simulink model "StateMachine2018b"  (R2018b)
settings: Solver=VariableStepAuto  StartTime=0.0  StopTime=10.0  RelTol=1e-3
settings Model: Creator=lenovo  LastModifiedBy=lenovo
settings DataIOCC: ReturnWorkspaceOutputs=on

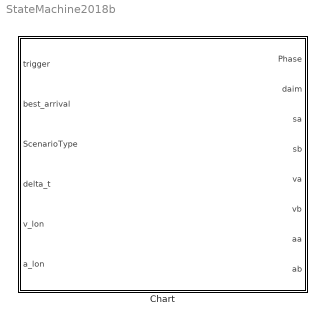
== system StateMachine2018b ==
  Chart : Stateflow chart  TreatAsAtomicUnit=on

== stateflow chart StateMachine2018b/Chart ==
  state initial
    en:
    sa = 0;
    sb = 40;
    va = 40/3.6;
    vb = 40/3.6;
    aa = 0;
    ab = 0;
    daim = 0;
    Phase = 0;
    du:
    Phase = 0;
    daim = 0;
    if (ScenarioType == 1)
    sa = 0;
    sb = 40;
    va = 40/3.6;
    vb = 40/3.6;
    aa = 0;
    ab = 0;
    else
    sa = -40;
    sb = 0;
    va = 40/3.6;
    vb = 40/3.6;
    aa = 0;
    ab = 0;
    end
  state phase1
    du:
    Phase = 1;
    sa = sa + delta_t * (va - v_lon) + 1/2 * (aa-a_lon) * delta_t^2;
    va = va + delta_t * aa;
    aa = 0;
    sb = sb + delta_t * (vb - v_lon)  + 1/2 * (ab-a_lon) * delta_t^2;
    vb = vb + delta_t * ab;
    ab = 0;
    daim = 1/2 * (sb - sa);
  state phase2
    du:
    Phase = 2;
    sa = sa + delta_t * (va - v_lon) + 1/2 * (aa-a_lon) * delta_t^2;
    va = va + delta_t * aa;
    aa = 0;
    sb = sb + delta_t * (vb - v_lon)  + 1/2 * (ab-a_lon) * delta_t^2;
    vb = vb + delta_t * ab;
    ab = 0;
    daim = 1/2 * (sb - sa);
  (default) -> initial
  initial -> phase1 : [trigger == 1]
  phase2 -> initial : [trigger == 0]
  phase1 -> phase2 : [best_arrival==1]
  data: trigger input double; Phase output double; best_arrival input double; ScenarioType input double; daim output double; sa output double; sb output double; va output double; vb output double; aa output double; ab output double; delta_t input double; v_lon input double; a_lon input double
